simulink model "semi_GSTA_const"  (R2018b)
settings: Solver=FixedStepAuto  StartTime=0.0  StopTime=30  FixedStep=0.01  RelTol=1e-3
InitFcn:
  | parameters_semi_gsta_const
model workspace: external: MAT-File (data not in the file)
values from neighbouring files (symbols this model uses):
  sample_time = 0.05    [parameters_semi_gsta_const.m]    (also in parameters_semi_gsta_vgain.m)
  x = [1.07906107302 2.04168763414 1.85257539652 1.93323325754 2.1580260637 1.75776173681 1.89939965925 1.8937988199 1.84120163561 1.64161458182 1.95451206586 1.46429138729 ... (9600 elements, 1600x6)]    [dat_x.mat]    (also in parameters_semi_gsta_const.m = [300   300    0.3    0.3]; parameters_semi_gsta_vgain.m = [2   2   0.05     5      1    0.3    0.3  1   0.5])
  x0 = 0.5    [parameters_semi_gsta_const.m]    (also in parameters_semi_gsta_vgain.m)
undefined symbols (not defined in the file or in its folder): fig_st, v0
libraries: sdolib x2
settings Model: Creator=DING  LastModifiedBy=DNN
settings SolverCC: ZeroCrossAlgorithm=Adaptive
settings OptimizationCC: DefaultParameterBehavior=Inlined  EnhancedBackFolding=on  PassReuseOutputArgsAs=Individual arguments  MaxStackSize=64  OptimizeBlockOrder=speed  DifferentSizesBufferReuse=on
settings DebuggingCC: IgnoredZcDiagnostic=none  ParameterTunabilityLossMsg=error
settings HardwareCC: ProdBitPerPointer=32  ProdBitPerSizeT=32  ProdBitPerPtrDiffT=32  ProdLargestAtomicInteger=Long  ProdLargestAtomicFloat=Double  ProdWordSize=32  ProdHWDeviceType=ARM Compatible->ARM 11
settings SFSimCC: MATLABDynamicMemAlloc=off
settings RTWCC: SystemTargetFile=ert.tlc  TemplateMakefile=ert_default_tmf  GenerateReport=on  Toolchain=Catkin  IncludeHyperlinkInReport=on  LaunchReport=on  GenerateTraceInfo=on  GenerateTraceReport=on  GenerateTraceReportSl=on  GenerateTraceReportSf=on  GenerateTraceReportEml=on
settings CodeAppCC: ForceParamTrailComments=on  IgnoreCustomStorageClasses=off  OperatorAnnotations=on  SimulinkDataObjDesc=on  SFDataObjDesc=on  InsertBlockDesc=on
settings ERTTargetCC: ERTCustomFileTemplate=example_file_process.tlc

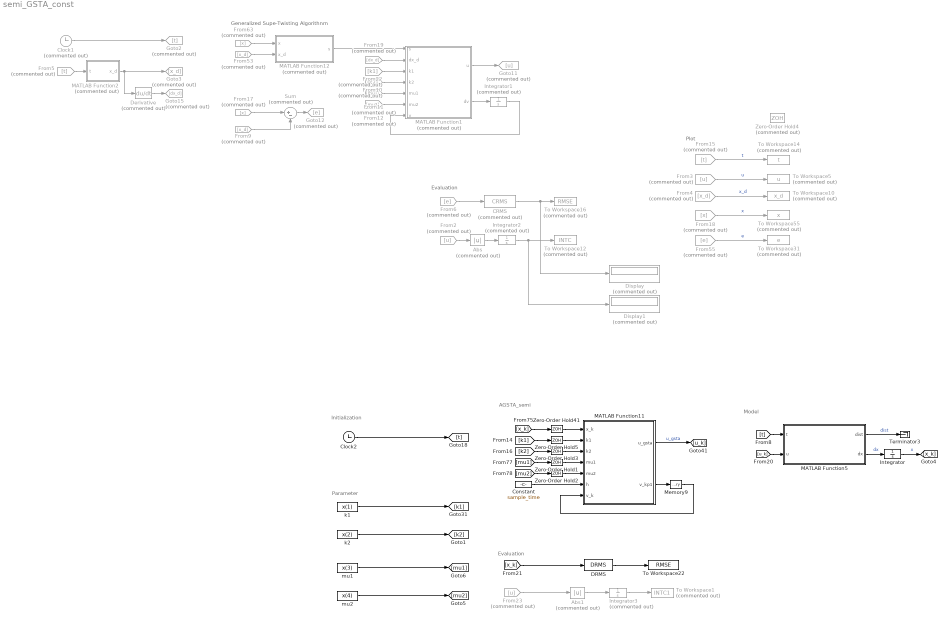
== system semi_GSTA_const ==
  note: AGSTA_semi
  note: Initialization
  note: Evaluation
  note: Parameter
  note: Plot
  note: Generalized Supe-Twisting Algorithnm
  note: Evaluation
  note: Model
  Abs : Abs  Commented=on
  Abs1 : Abs  Commented=on
  CRMS : sdolib/RMS Blocks/CRMS  Commented=on
      settings: SourceProductBaseCode=SO
  Clock1 : Clock  Commented=on
  Clock2 : Clock
  Constant : Constant  Value=sample_time  SampleTime=sample_time
  DRMS : sdolib/RMS Blocks/DRMS  Ts=sample_time
      settings: SourceProductBaseCode=SO
  Derivative : Derivative  Commented=on
  Display : Display  Commented=on
  Display1 : Display  Commented=on
  From10 : From  Commented=on  GotoTag=k2
  From11 : From  Commented=on  GotoTag=mu1
  From12 : From  Commented=on  GotoTag=mu2
  From15 : From  Commented=on  GotoTag=t
  From17 : From  Commented=on  GotoTag=x
  From18 : From  Commented=on  GotoTag=x
  From19 : From  Commented=on  GotoTag=dx_d
  From2 : From  Commented=on  GotoTag=u
  From22 : From  Commented=on  GotoTag=k1
  From23 : From  Commented=on  GotoTag=u
  From3 : From  Commented=on  GotoTag=u
  From4 : From  Commented=on  GotoTag=x_d
  From5 : From  Commented=on  GotoTag=t
  From53 : From  Commented=on  GotoTag=x_d
  From55 : From  Commented=on  GotoTag=e
  From6 : From  Commented=on  GotoTag=e
  From63 : From  Commented=on  GotoTag=x
  From9 : From  Commented=on  GotoTag=x_d
  Goto11 : Goto  Commented=on  GotoTag=u
  Goto12 : Goto  Commented=on  GotoTag=e
  Goto15 : Goto  Commented=on  GotoTag=dx_d
  Goto2 : Goto  Commented=on  GotoTag=t
  Goto3 : Goto  Commented=on  GotoTag=x_d
  Integrator : Integrator  InitialCondition=x0
  Integrator1 : Integrator  Commented=on  InitialCondition=v0
  Integrator2 : Integrator  Commented=on  InitialCondition=v0
  Integrator3 : Integrator  Commented=on  InitialCondition=v0
  MATLAB Function1 : MATLAB Function  Commented=on  TreatAsAtomicUnit=on
  MATLAB Function11 : MATLAB Function  TreatAsAtomicUnit=on
  MATLAB Function12 : MATLAB Function  Commented=on  TreatAsAtomicUnit=on
  MATLAB Function2 : MATLAB Function  Commented=on  TreatAsAtomicUnit=on
  MATLAB Function5 : MATLAB Function  TreatAsAtomicUnit=on
  Memory9 : Memory  InheritSampleTime=on
  Sum : Sum  Commented=on  Inputs=|+-
  Terminator3 : Terminator
  To Workspace1 : ToWorkspace  Commented=on  VariableName=INTC1  SampleTime=-1
      settings: MaxDataPoints=1
  To Workspace10 : ToWorkspace  Commented=on  VariableName=x_d  SampleTime=-1
  To Workspace12 : ToWorkspace  Commented=on  VariableName=INTC  SampleTime=-1
      settings: MaxDataPoints=1
  To Workspace14 : ToWorkspace  Commented=on  VariableName=t  SampleTime=-1
  To Workspace16 : ToWorkspace  Commented=on  VariableName=RMSE  SampleTime=-1
      settings: MaxDataPoints=1
  To Workspace22 : ToWorkspace  VariableName=RMSE  SampleTime=-1
      settings: MaxDataPoints=1
  To Workspace31 : ToWorkspace  Commented=on  VariableName=e  SampleTime=-1
  To Workspace5 : ToWorkspace  Commented=on  VariableName=u  SampleTime=-1
  To Workspace55 : ToWorkspace  Commented=on  VariableName=x  SampleTime=-1
  Zero-Order Hold{1..3,5,41} (5 alike) : ZeroOrderHold  SampleTime=sample_time
  Zero-Order Hold4 : ZeroOrderHold  Commented=on  SampleTime=fig_st
  k1 : Constant  Value=x(1)
  k2 : Constant  Value=x(2)
  mu1 : Constant  Value=x(3)
  mu2 : Constant  Value=x(4)
  wires:
  Clock2/1 -> [t]
  [mu1] -> Zero-Order Hold1/1
  [mu2] -> Zero-Order Hold2/1
  MATLAB Function11/2(v_kp1) -> Memory9/1
  Memory9/1 -> MATLAB Function11/7(v_k)
  Constant/1 -> MATLAB Function11/6(h)
  Zero-Order Hold1/1 -> MATLAB Function11/4(mu1)
  Zero-Order Hold2/1 -> MATLAB Function11/5(mu2)
  MATLAB Function11/1(u_gsta) -> [u_k]  "u_gsta"
  Abs/1 -> Integrator2/1
  From11/1 -> MATLAB Function1/5(mu1)
  Clock1/1 -> Goto2/1
  From10/1 -> MATLAB Function1/4(k2)
  From22/1 -> MATLAB Function1/3(k1)
  From18/1 -> To Workspace55/1  "x"
  From19/1 -> MATLAB Function1/2(dx_d)
  From17/1 -> Sum/1
  Derivative/1 -> Goto15/1
  Sum/1 -> Goto12/1
  From63/1 -> MATLAB Function12/1(x)
  From12/1 -> MATLAB Function1/6(mu2)
  From15/1 -> To Workspace14/1  "t"
  Integrator2/1 -> To Workspace12/1, Display1/1
  MATLAB Function1/1(u) -> Goto11/1
  From4/1 -> To Workspace10/1  "x_d"
  From5/1 -> MATLAB Function2/1(t)
  From55/1 -> To Workspace31/1  "e"
  From2/1 -> Abs/1
  MATLAB Function2/1(x_d) -> Goto3/1, Derivative/1
  CRMS/1 -> To Workspace16/1, Display/1
  From6/1 -> CRMS/1
  Integrator1/1 -> MATLAB Function1/7(v)
  From3/1 -> To Workspace5/1  "u"
  MATLAB Function1/2(dv) -> Integrator1/1
  From9/1 -> Sum/2
  MATLAB Function12/1(s) -> MATLAB Function1/1(s)
  From53/1 -> MATLAB Function12/2(x_d)
  [t] -> MATLAB Function5/1(t)
  Integrator/1 -> [x_k]  "x"
  MATLAB Function5/2(dx) -> Integrator/1  "dx"
  MATLAB Function5/1(dist) -> Terminator3/1  "dist"
  [u_k] -> MATLAB Function5/2(u)
  Zero-Order Hold3/1 -> MATLAB Function11/3(k2)
  Zero-Order Hold5/1 -> MATLAB Function11/2(k1)
  [k1] -> Zero-Order Hold5/1
  [k2] -> Zero-Order Hold3/1
  k1/1 -> [k1]
  k2/1 -> [k2]
  mu2/1 -> [mu2]
  mu1/1 -> [mu1]
  From23/1 -> Abs1/1
  Integrator3/1 -> To Workspace1/1
  Abs1/1 -> Integrator3/1
  [x_k] -> DRMS/1
  DRMS/1 -> To Workspace22/1
  Zero-Order Hold41/1 -> MATLAB Function11/1(x_k)
  [x_k] -> Zero-Order Hold41/1

== matlab function semi_GSTA_const/MATLAB Function2 ==
  data: x_d output; t input
function x_d= desired(t)

x_d=sin(0.8*t)+cos(t);

end

== matlab function semi_GSTA_const/MATLAB Function5 ==
  data: dist output; dx output; t input; u input
function [dist,dx]= Dynamic_Model(t,u)

% fx=0.6*sin(x)+0.7*x^2-1.5*x;
% dxt=0.8*cos(x)*x+0.05*cos(3*t)+0.08*sin(t);
% dx=fx+dxt+u;

dist=5*cos(t);
dx=u+dist;

end

== matlab function semi_GSTA_const/MATLAB Function11 ==
  data: x_k input; k1 input; k2 input; mu1 input; mu2 input; h input; v_k input; u_gsta output; v_kp1 output
function [u_gsta, v_kp1] = GSTA(x_k, k1, k2, mu1, mu2, h, v_k)

lam_sum = - k1 * (mu1 * abs(x_k) ^ - 0.5 + mu2);
lam_multi = k2 * (0.5 * mu1 * abs(x_k) ^ - 1 + 1.5 * mu1 * mu2 * abs(x_k) ^ - 0.5 + mu2 ^ 2 );

if x_k == 0
        q_sum = 0;
        q_multi = 0;
else
        q_sum = (2 - h * lam_sum ) / (1 - h * lam_sum + h ^ 2 * lam_multi ); 
        q_multi = 1 / (1 - h * lam_sum + h ^ 2 * lam_multi );
end

u1_k = q_sum - 1;    % u1_k=q1+q2-1;
u2_k = 1 / h * (u1_k - q_multi);   % u2_k=1/h*(u1_k-q1*q2);


v_kp1 = v_k + u2_k * x_k;
u_gsta = 1 / h * ( - x_k + u1_k * x_k ) + v_kp1;

end

== matlab function semi_GSTA_const/MATLAB Function1 ==
  data: s input; dx_d input; u output; dv output; k1 input; k2 input; mu1 input; mu2 input; v input
function [u,dv] = GSTA(s,dx_d,k1,k2,mu1,mu2,v)

fa_1s=mu1*abs(s)^0.5*sign(s)+mu2*s;
fa_2s=0.5*mu1^2*sign(s)+1.5*mu1*mu2*abs(s)^0.5*sign(s)+mu2^2*s;
dv=-k2*fa_2s;
u=dx_d-k1*fa_1s+v;

end

== matlab function semi_GSTA_const/MATLAB Function12 ==
  data: x input; x_d input; s output
function s = sliding_face(x,x_d)

s=x-x_d;

end
